simulink model "Fload"  (R2022a)
settings: Solver=FixedStepDiscrete  StartTime=0.0  StopTime=10.0  RelTol=1e-3  EnableMultiTasking=on
InitFcn:
  | test_init
settings Model: Creator=highi  LastModifiedBy=highi
settings HardwareCC: ProdBitPerPointer=32  ProdBitPerSizeT=32  ProdBitPerPtrDiffT=32  ProdLargestAtomicFloat=None  ProdIntDivRoundTo=Undefined  ProdEndianess=Unspecified  ProdWordSize=32  ProdHWDeviceType=ASIC/FPGA->ASIC/FPGA  TargetBitPerPointer=64  TargetBitPerSizeT=64  TargetBitPerPtrDiffT=64  TargetLongLongMode=on  TargetIntDivRoundTo=Zero  TargetEndianess=LittleEndian  TargetWordSize=64  TargetHWDeviceType=Custom Processor->MATLAB Host Computer  ProdEqTarget=off

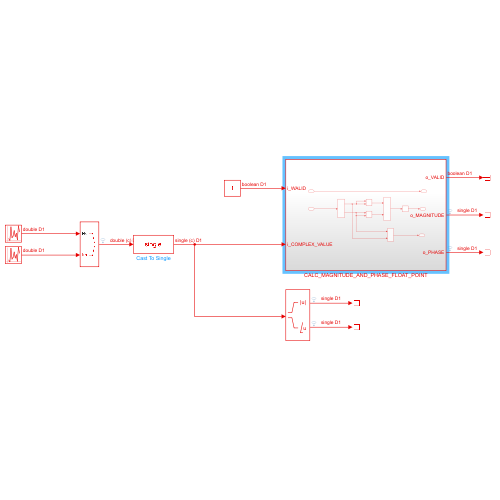
[thumbnail: Simulink's stored preview of the top-level diagram]
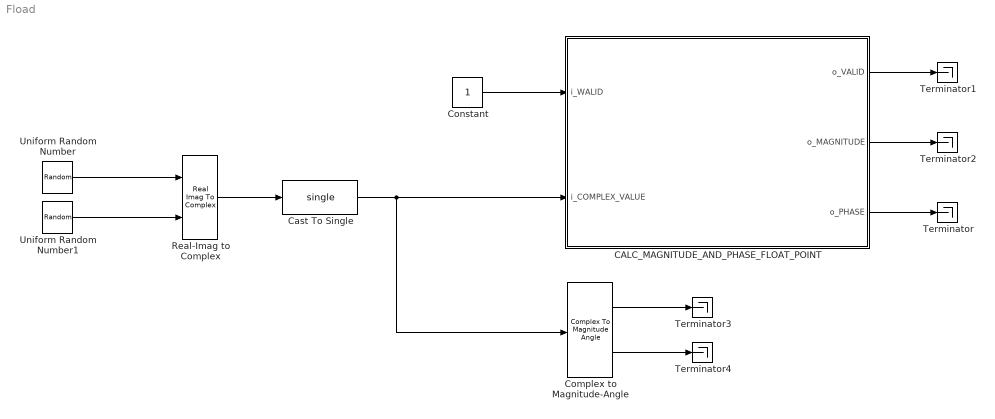
== system Fload ==
  CALC_MAGNITUDE_AND_PHASE_FLOAT_POINT : Subsystem
  Cast To Single : DataTypeConversion  OutDataTypeStr=single  SaturateOnIntegerOverflow=off  RndMeth=Floor
  Complex to Magnitude-Angle : ComplexToMagnitudeAngle
  Constant : Constant  OutDataTypeStr=boolean  SampleTime=1
  Real-Imag to Complex : RealImagToComplex
  Terminator{,1..4} (5 alike) : Terminator
  Uniform Random Number : UniformRandomNumber  Minimum=0  Maximum=2097151.49999809265  Seed=21  SampleTime=1
  Uniform Random Number1 : UniformRandomNumber  Minimum=0  Maximum=2097151.49999809265  Seed=22  SampleTime=1
  wires:
  Uniform Random Number1/1 -> Real-Imag to Complex/2
  Uniform Random Number/1 -> Real-Imag to Complex/1
  Real-Imag to Complex/1 -> Cast To Single/1
  Cast To Single/1 -> CALC_MAGNITUDE_AND_PHASE_FLOAT_POINT/2(i_COMPLEX_VALUE), Complex to Magnitude-Angle/1
  Constant/1 -> CALC_MAGNITUDE_AND_PHASE_FLOAT_POINT/1(i_WALID)
  CALC_MAGNITUDE_AND_PHASE_FLOAT_POINT/3(o_PHASE) -> Terminator/1
  CALC_MAGNITUDE_AND_PHASE_FLOAT_POINT/2(o_MAGNITUDE) -> Terminator2/1
  CALC_MAGNITUDE_AND_PHASE_FLOAT_POINT/1(o_VALID) -> Terminator1/1
  Complex to Magnitude-Angle/2 -> Terminator4/1
  Complex to Magnitude-Angle/1 -> Terminator3/1

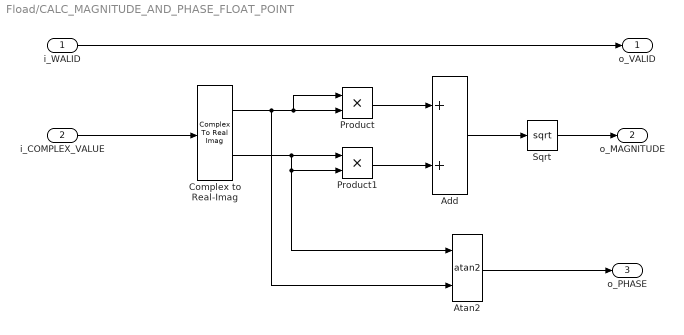
== system Fload/CALC_MAGNITUDE_AND_PHASE_FLOAT_POINT ==
  i_WALID : Inport
  i_COMPLEX_VALUE : Inport  Port=2
  Add : Sum
  Atan2 : Trigonometry  Operator=atan2
  Complex to Real-Imag : ComplexToRealImag
  Product : Product
  Product1 : Product
  Sqrt : Sqrt
  o_VALID : Outport
  o_MAGNITUDE : Outport  Port=2
  o_PHASE : Outport  Port=3
  wires:
  Complex to Real-Imag/2 -> Product1/2, Atan2/1, Product1/1
  Complex to Real-Imag/1 -> Atan2/2, Product/1, Product/2
  Product1/1 -> Add/2
  Add/1 -> Sqrt/1
  Product/1 -> Add/1
  i_COMPLEX_VALUE/1 -> Complex to Real-Imag/1
  Atan2/1 -> o_PHASE/1
  Sqrt/1 -> o_MAGNITUDE/1
  i_WALID/1 -> o_VALID/1
